simulink library "tqr"  (R2021b)
settings: Solver=VariableStepAuto  StartTime=0.0  StopTime=10.0  RelTol=1e-3
undefined symbols (not defined in the file or in its folder): ATQR_AltRDCActiveFEDUInc_X_pct, ATQR_AltRDCActiveFEDUInc_Y_enum, ATQR_AltRDCActiveFEDUTs_X_pct, ATQR_AltRDCActiveFEDUTs_Y_enum, ATQR_AltRDCActiveREDUInc_X_pct, ATQR_AltRDCActiveREDUInc_Y_enum, ATQR_AltRDCActiveREDUTs_X_pct, ATQR_AltRDCActiveREDUTs_Y_enum, ATQR_CreepFEDUTqIncSR_X_rpm, ATQR_CreepFEDUTqIncSR_Y_Nm, ATQR_CreepFEDUTs_X_rpm, ATQR_CreepFEDUTs_Y_Nm, ATQR_EcoTqFrIncGain_X_Nm, ATQR_EcoTqFrIncGain_Y_pct, ATQR_EcoTqRrIncGain_X_Nm, ATQR_EcoTqRrIncGain_Y_pct, ATQR_EL1FEDUTqDecSR_Y_Nm, ATQR_EL1FEDUTqIncSR_X_rpm, ATQR_EL1FEDUTqIncSR_Y_pct, ATQR_EL1FEDUTs_X_rpm, ATQR_EL1FEDUTs_Y_Nm, ATQR_EL1REDUTqDecSR_Y_Nm, ATQR_EL1REDUTs_Y_Nm, ATQR_FEDUEL1RegenTs_X_rpm, ATQR_FEDUTIPOutTs_X_rpm, ATQR_FrNegRateLimitIncN_X_rpm, ATQR_FrNegRateLimitIncN_Y_Nm, ATQR_FrPosRateLimitIncN_X_rpm, ATQR_FrPosRateLimitIncN_Y_Nm, ATQR_FShaftSpdTqLimCoe_X_rpm, ATQR_FTimerTqLimCoe_X_s, ATQR_FTqZeroTransUpBoundN_X_rpm, ATQR_NL1FEDUTqDecSR_Y_Nm, ATQR_NL1FEDUTqIncSR_X_rpm, ATQR_NL1FEDUTqIncSR_Y_pct, ATQR_NL1FEDUTs_X_rpm, ATQR_NL1FEDUTs_Y_Nm, ATQR_NL1REDUTqDecSR_Y_Nm, ATQR_NL1REDUTs_Y_Nm, ATQR_NormalTqFrIncGain_X_Nm, ATQR_NormalTqFrIncGain_Y_pct, ATQR_NormalTqRrIncGain_X_Nm, ATQR_NormalTqRrIncGain_Y_pct, ATQR_RrNegRateLimitIncN_X_rpm, ATQR_RrNegRateLimitIncN_Y_Nm, ATQR_RrPosRateLimitIncN_X_rpm, ATQR_RrPosRateLimitIncN_Y_Nm, ATQR_RShaftSpdTqLimCoe_X_rpm, ATQR_RTimerTqLimCoe_X_s, ATQR_SL1FEDUTqDecSR_Y_Nm, ATQR_SL1FEDUTqIncSR_X_rpm, ATQR_SL1FEDUTqIncSR_Y_pct, ATQR_SL1FEDUTs_X_rpm, ATQR_SL1FEDUTs_Y_Nm, ATQR_SL1REDUTqDecSR_Y_Nm, ATQR_SL1REDUTs_Y_Nm, ATQR_SportTqFrIncGain_X_Nm, ATQR_SportTqFrIncGain_Y_pct, ATQR_SportTqRrIncGain_X_Nm, ATQR_SportTqRrIncGain_Y_pct ... (+269)
libraries: hcu_lib x15, simulink x13, $bdroot x3
(part 9 of 9)

== system tqr/TQR/Determine Torque Request/TorqueArbitrament/TorqueSmooth/Rear wheel rate limit determination/VTQR_ECOREDURateLimitInc_Nm/LV4 ==
  VDHP_ActAPSPosn_pct : Inport
  VTQD_TqTargetShaftSpd_rpm : Inport  Port=2
  VTQR_EcoTqRrIncGain_c : Inport  Port=3
  Action Port : ActionPort
  MTQR_EL4REDUTqIncSR_Z_Nm : Lookup_n-D  BreakpointsForDimension1=ATQR_EL1FEDUTqIncSR_Y_pct  BreakpointsForDimension2=ATQR_EL1FEDUTqIncSR_X_rpm  Table=MTQR_EL4REDUTqIncSR_Z_Nm  ExtrapMethod=Clip  InternalRulePriority=Speed  RndMeth=Simplest  InputSameDT=on
      settings: InputPortMap=u0,u1
  Product : Product
  VTQR_EL4REDUTqIncSR_Nm : Outport
  wires:
  VDHP_ActAPSPosn_pct/1 -> MTQR_EL4REDUTqIncSR_Z_Nm/1
  VTQD_TqTargetShaftSpd_rpm/1 -> MTQR_EL4REDUTqIncSR_Z_Nm/2
  VTQR_EcoTqRrIncGain_c/1 -> Product/2
  MTQR_EL4REDUTqIncSR_Z_Nm/1 -> Product/1
  Product/1 -> VTQR_EL4REDUTqIncSR_Nm/1

== system tqr/TQR/Determine Torque Request/TorqueArbitrament/TorqueSmooth/Rear wheel rate limit determination/VTQR_ECOREDURateLimitInc_Nm/LV5 ==
  VDHP_ActAPSPosn_pct : Inport
  VTQD_TqTargetShaftSpd_rpm : Inport  Port=2
  VTQR_EcoTqRrIncGain_c : Inport  Port=3
  Action Port : ActionPort
  MTQR_EL5REDUTqIncSR_Z_Nm : Lookup_n-D  BreakpointsForDimension1=ATQR_EL1FEDUTqIncSR_Y_pct  BreakpointsForDimension2=ATQR_EL1FEDUTqIncSR_X_rpm  Table=MTQR_EL5REDUTqIncSR_Z_Nm  ExtrapMethod=Clip  InternalRulePriority=Speed  RndMeth=Simplest  InputSameDT=on
      settings: InputPortMap=u0,u1
  Product : Product
  VTQR_EL5REDUTqIncSR_Nm : Outport
  wires:
  VDHP_ActAPSPosn_pct/1 -> MTQR_EL5REDUTqIncSR_Z_Nm/1
  VTQD_TqTargetShaftSpd_rpm/1 -> MTQR_EL5REDUTqIncSR_Z_Nm/2
  VTQR_EcoTqRrIncGain_c/1 -> Product/2
  MTQR_EL5REDUTqIncSR_Z_Nm/1 -> Product/1
  Product/1 -> VTQR_EL5REDUTqIncSR_Nm/1

== system tqr/TQR/Determine Torque Request/TorqueArbitrament/TorqueSmooth/Rear wheel rate limit determination/VTQR_ECOREDURateLimitInc_Nm/OPD ==
  VDHP_ActAPSPosn_pct : Inport
  VTQD_TqTargetShaftSpd_rpm : Inport  Port=2
  VTQR_EcoTqRrIncGain_c : Inport  Port=3
  Action Port : ActionPort
  MTQR_EOPDREDUTqIncSR_Z_Nm : Lookup_n-D  BreakpointsForDimension1=ATQR_EL1FEDUTqIncSR_Y_pct  BreakpointsForDimension2=ATQR_EL1FEDUTqIncSR_X_rpm  Table=MTQR_EOPDREDUTqIncSR_Z_Nm  ExtrapMethod=Clip  InternalRulePriority=Speed  RndMeth=Simplest  InputSameDT=on
      settings: InputPortMap=u0,u1
  Product : Product
  VTQR_EOPDREDUTqIncSR_Nm : Outport
  wires:
  VDHP_ActAPSPosn_pct/1 -> MTQR_EOPDREDUTqIncSR_Z_Nm/1
  VTQD_TqTargetShaftSpd_rpm/1 -> MTQR_EOPDREDUTqIncSR_Z_Nm/2
  VTQR_EcoTqRrIncGain_c/1 -> Product/2
  MTQR_EOPDREDUTqIncSR_Z_Nm/1 -> Product/1
  Product/1 -> VTQR_EOPDREDUTqIncSR_Nm/1

== system tqr/TQR/Determine Torque Request/TorqueArbitrament/TorqueSmooth/Rear wheel rate limit determination/VTQR_NORMALREDURateLimitDec_Nm/Invalid ==
  VTQR_REDUWhlTqReqSmoothDelay_Nm : Inport
  VTQD_TqTargetShaftSpd_rpm : Inport  Port=2
  Action Port : ActionPort
  MTQR_NL1REDUTqDecSR_Z_Nm : Lookup_n-D  BreakpointsForDimension1=ATQR_NL1REDUTqDecSR_Y_Nm  BreakpointsForDimension2=ATQR_NL1FEDUTqIncSR_X_rpm  Table=MTQR_NL1REDUTqDecSR_Z_Nm  ExtrapMethod=Clip  InternalRulePriority=Speed  RndMeth=Simplest  InputSameDT=on
      settings: InputPortMap=u0,u1
  VTQR_NL1REDUTqDecSR_Nm : Outport
  wires:
  VTQD_TqTargetShaftSpd_rpm/1 -> MTQR_NL1REDUTqDecSR_Z_Nm/2
  MTQR_NL1REDUTqDecSR_Z_Nm/1 -> VTQR_NL1REDUTqDecSR_Nm/1
  VTQR_REDUWhlTqReqSmoothDelay_Nm/1 -> MTQR_NL1REDUTqDecSR_Z_Nm/1

== system tqr/TQR/Determine Torque Request/TorqueArbitrament/TorqueSmooth/Rear wheel rate limit determination/VTQR_NORMALREDURateLimitDec_Nm/LV1 ==
  VTQR_REDUWhlTqReqSmoothDelay_Nm : Inport
  VTQD_TqTargetShaftSpd_rpm : Inport  Port=2
  Action Port : ActionPort
  MTQR_NL1REDUTqDecSR_Z_Nm : Lookup_n-D  BreakpointsForDimension1=ATQR_NL1REDUTqDecSR_Y_Nm  BreakpointsForDimension2=ATQR_NL1FEDUTqIncSR_X_rpm  Table=MTQR_NL1REDUTqDecSR_Z_Nm  ExtrapMethod=Clip  InternalRulePriority=Speed  RndMeth=Simplest  InputSameDT=on
      settings: InputPortMap=u0,u1
  VTQR_NL1REDUTqDecSR_Nm : Outport
  wires:
  VTQR_REDUWhlTqReqSmoothDelay_Nm/1 -> MTQR_NL1REDUTqDecSR_Z_Nm/1
  MTQR_NL1REDUTqDecSR_Z_Nm/1 -> VTQR_NL1REDUTqDecSR_Nm/1
  VTQD_TqTargetShaftSpd_rpm/1 -> MTQR_NL1REDUTqDecSR_Z_Nm/2

== system tqr/TQR/Determine Torque Request/TorqueArbitrament/TorqueSmooth/Rear wheel rate limit determination/VTQR_NORMALREDURateLimitDec_Nm/LV2 ==
  VTQR_REDUWhlTqReqSmoothDelay_Nm : Inport
  VTQD_TqTargetShaftSpd_rpm : Inport  Port=2
  Action Port : ActionPort
  MTQR_NL2REDUTqDecSR_Z_Nm : Lookup_n-D  BreakpointsForDimension1=ATQR_NL1REDUTqDecSR_Y_Nm  BreakpointsForDimension2=ATQR_NL1FEDUTqIncSR_X_rpm  Table=MTQR_NL2REDUTqDecSR_Z_Nm  ExtrapMethod=Clip  InternalRulePriority=Speed  RndMeth=Simplest  InputSameDT=on
      settings: InputPortMap=u0,u1
  VTQR_NL2REDUTqDecSR_Nm : Outport
  wires:
  MTQR_NL2REDUTqDecSR_Z_Nm/1 -> VTQR_NL2REDUTqDecSR_Nm/1
  VTQR_REDUWhlTqReqSmoothDelay_Nm/1 -> MTQR_NL2REDUTqDecSR_Z_Nm/1
  VTQD_TqTargetShaftSpd_rpm/1 -> MTQR_NL2REDUTqDecSR_Z_Nm/2

== system tqr/TQR/Determine Torque Request/TorqueArbitrament/TorqueSmooth/Rear wheel rate limit determination/VTQR_NORMALREDURateLimitDec_Nm/LV3 ==
  VTQR_REDUWhlTqReqSmoothDelay_Nm : Inport
  VTQD_TqTargetShaftSpd_rpm : Inport  Port=2
  Action Port : ActionPort
  MTQR_NL3REDUTqDecSR_Z_Nm : Lookup_n-D  BreakpointsForDimension1=ATQR_NL1REDUTqDecSR_Y_Nm  BreakpointsForDimension2=ATQR_NL1FEDUTqIncSR_X_rpm  Table=MTQR_NL3REDUTqDecSR_Z_Nm  ExtrapMethod=Clip  InternalRulePriority=Speed  RndMeth=Simplest  InputSameDT=on
      settings: InputPortMap=u0,u1
  VTQR_NL3REDUTqDecSR_Nm : Outport
  wires:
  VTQR_REDUWhlTqReqSmoothDelay_Nm/1 -> MTQR_NL3REDUTqDecSR_Z_Nm/1
  VTQD_TqTargetShaftSpd_rpm/1 -> MTQR_NL3REDUTqDecSR_Z_Nm/2
  MTQR_NL3REDUTqDecSR_Z_Nm/1 -> VTQR_NL3REDUTqDecSR_Nm/1

== system tqr/TQR/Determine Torque Request/TorqueArbitrament/TorqueSmooth/Rear wheel rate limit determination/VTQR_NORMALREDURateLimitDec_Nm/LV4 ==
  VTQR_REDUWhlTqReqSmoothDelay_Nm : Inport
  VTQD_TqTargetShaftSpd_rpm : Inport  Port=2
  Action Port : ActionPort
  MTQR_NL4REDUTqDecSR_Z_Nm : Lookup_n-D  BreakpointsForDimension1=ATQR_NL1REDUTqDecSR_Y_Nm  BreakpointsForDimension2=ATQR_NL1FEDUTqIncSR_X_rpm  Table=MTQR_NL4REDUTqDecSR_Z_Nm  ExtrapMethod=Clip  InternalRulePriority=Speed  RndMeth=Simplest  InputSameDT=on
      settings: InputPortMap=u0,u1
  VTQR_NL4REDUTqDecSR_Nm : Outport
  wires:
  VTQR_REDUWhlTqReqSmoothDelay_Nm/1 -> MTQR_NL4REDUTqDecSR_Z_Nm/1
  VTQD_TqTargetShaftSpd_rpm/1 -> MTQR_NL4REDUTqDecSR_Z_Nm/2
  MTQR_NL4REDUTqDecSR_Z_Nm/1 -> VTQR_NL4REDUTqDecSR_Nm/1

== system tqr/TQR/Determine Torque Request/TorqueArbitrament/TorqueSmooth/Rear wheel rate limit determination/VTQR_NORMALREDURateLimitDec_Nm/LV5 ==
  VTQR_REDUWhlTqReqSmoothDelay_Nm : Inport
  VTQD_TqTargetShaftSpd_rpm : Inport  Port=2
  Action Port : ActionPort
  MTQR_NL5REDUTqDecSR_Z_Nm : Lookup_n-D  BreakpointsForDimension1=ATQR_NL1REDUTqDecSR_Y_Nm  BreakpointsForDimension2=ATQR_NL1FEDUTqIncSR_X_rpm  Table=MTQR_NL5REDUTqDecSR_Z_Nm  ExtrapMethod=Clip  InternalRulePriority=Speed  RndMeth=Simplest  InputSameDT=on
      settings: InputPortMap=u0,u1
  VTQR_NL5REDUTqDecSR_Nm : Outport
  wires:
  VTQR_REDUWhlTqReqSmoothDelay_Nm/1 -> MTQR_NL5REDUTqDecSR_Z_Nm/1
  VTQD_TqTargetShaftSpd_rpm/1 -> MTQR_NL5REDUTqDecSR_Z_Nm/2
  MTQR_NL5REDUTqDecSR_Z_Nm/1 -> VTQR_NL5REDUTqDecSR_Nm/1

== system tqr/TQR/Determine Torque Request/TorqueArbitrament/TorqueSmooth/Rear wheel rate limit determination/VTQR_NORMALREDURateLimitDec_Nm/OPD ==
  VTQR_REDUWhlTqReqSmoothDelay_Nm : Inport
  VTQD_TqTargetShaftSpd_rpm : Inport  Port=2
  Action Port : ActionPort
  MTQR_NOPDREDUTqDecSR_Z_Nm : Lookup_n-D  BreakpointsForDimension1=ATQR_NL1REDUTqDecSR_Y_Nm  BreakpointsForDimension2=ATQR_NL1FEDUTqIncSR_X_rpm  Table=MTQR_NOPDREDUTqDecSR_Z_Nm  ExtrapMethod=Clip  InternalRulePriority=Speed  RndMeth=Simplest  InputSameDT=on
      settings: InputPortMap=u0,u1
  VTQR_NOPDREDUTqDecSR_Nm : Outport
  wires:
  VTQR_REDUWhlTqReqSmoothDelay_Nm/1 -> MTQR_NOPDREDUTqDecSR_Z_Nm/1
  VTQD_TqTargetShaftSpd_rpm/1 -> MTQR_NOPDREDUTqDecSR_Z_Nm/2
  MTQR_NOPDREDUTqDecSR_Z_Nm/1 -> VTQR_NOPDREDUTqDecSR_Nm/1

== system tqr/TQR/Determine Torque Request/TorqueArbitrament/TorqueSmooth/Rear wheel rate limit determination/VTQR_NORMALREDURateLimitInc_Nm/Invalid ==
  VDHP_ActAPSPosn_pct : Inport
  VTQD_TqTargetShaftSpd_rpm : Inport  Port=2
  Action Port : ActionPort
  MTQR_NL1REDUTqIncSR_Z_Nm : Lookup_n-D  BreakpointsForDimension1=ATQR_NL1FEDUTqIncSR_Y_pct  BreakpointsForDimension2=ATQR_NL1FEDUTqIncSR_X_rpm  Table=MTQR_NL1REDUTqIncSR_Z_Nm  ExtrapMethod=Clip  InternalRulePriority=Speed  RndMeth=Simplest  InputSameDT=on
      settings: InputPortMap=u0,u1
  VTQR_NL1REDUTqIncSR_Nm : Outport
  wires:
  VTQD_TqTargetShaftSpd_rpm/1 -> MTQR_NL1REDUTqIncSR_Z_Nm/2
  MTQR_NL1REDUTqIncSR_Z_Nm/1 -> VTQR_NL1REDUTqIncSR_Nm/1
  VDHP_ActAPSPosn_pct/1 -> MTQR_NL1REDUTqIncSR_Z_Nm/1

== system tqr/TQR/Determine Torque Request/TorqueArbitrament/TorqueSmooth/Rear wheel rate limit determination/VTQR_NORMALREDURateLimitInc_Nm/LV1 ==
  VDHP_ActAPSPosn_pct : Inport
  VTQD_TqTargetShaftSpd_rpm : Inport  Port=2
  VTQR_NormalTqRrIncGain_c : Inport  Port=3
  Action Port : ActionPort
  MTQR_NL1REDUTqIncSR_Z_Nm : Lookup_n-D  BreakpointsForDimension1=ATQR_NL1FEDUTqIncSR_Y_pct  BreakpointsForDimension2=ATQR_NL1FEDUTqIncSR_X_rpm  Table=MTQR_NL1REDUTqIncSR_Z_Nm  ExtrapMethod=Clip  InternalRulePriority=Speed  RndMeth=Simplest  InputSameDT=on
      settings: InputPortMap=u0,u1
  Product : Product
  VTQR_NL1REDUTqIncSR_Nm : Outport
  wires:
  VDHP_ActAPSPosn_pct/1 -> MTQR_NL1REDUTqIncSR_Z_Nm/1
  VTQD_TqTargetShaftSpd_rpm/1 -> MTQR_NL1REDUTqIncSR_Z_Nm/2
  MTQR_NL1REDUTqIncSR_Z_Nm/1 -> Product/1
  Product/1 -> VTQR_NL1REDUTqIncSR_Nm/1
  VTQR_NormalTqRrIncGain_c/1 -> Product/2

== system tqr/TQR/Determine Torque Request/TorqueArbitrament/TorqueSmooth/Rear wheel rate limit determination/VTQR_NORMALREDURateLimitInc_Nm/LV2 ==
  VDHP_ActAPSPosn_pct : Inport
  VTQD_TqTargetShaftSpd_rpm : Inport  Port=2
  VTQR_NormalTqRrIncGain_c : Inport  Port=3
  Action Port : ActionPort
  MTQR_NL2REDUTqIncSR_Z_Nm : Lookup_n-D  BreakpointsForDimension1=ATQR_NL1FEDUTqIncSR_Y_pct  BreakpointsForDimension2=ATQR_NL1FEDUTqIncSR_X_rpm  Table=MTQR_NL2REDUTqIncSR_Z_Nm  ExtrapMethod=Clip  InternalRulePriority=Speed  RndMeth=Simplest  InputSameDT=on
      settings: InputPortMap=u0,u1
  Product : Product
  VTQR_NL2REDUTqIncSR_Nm : Outport
  wires:
  VDHP_ActAPSPosn_pct/1 -> MTQR_NL2REDUTqIncSR_Z_Nm/1
  VTQD_TqTargetShaftSpd_rpm/1 -> MTQR_NL2REDUTqIncSR_Z_Nm/2
  Product/1 -> VTQR_NL2REDUTqIncSR_Nm/1
  MTQR_NL2REDUTqIncSR_Z_Nm/1 -> Product/1
  VTQR_NormalTqRrIncGain_c/1 -> Product/2

== system tqr/TQR/Determine Torque Request/TorqueArbitrament/TorqueSmooth/Rear wheel rate limit determination/VTQR_NORMALREDURateLimitInc_Nm/LV3 ==
  VDHP_ActAPSPosn_pct : Inport
  VTQD_TqTargetShaftSpd_rpm : Inport  Port=2
  VTQR_NormalTqRrIncGain_c : Inport  Port=3
  Action Port : ActionPort
  MTQR_NL3REDUTqIncSR_Z_Nm : Lookup_n-D  BreakpointsForDimension1=ATQR_NL1FEDUTqIncSR_Y_pct  BreakpointsForDimension2=ATQR_NL1FEDUTqIncSR_X_rpm  Table=MTQR_NL3REDUTqIncSR_Z_Nm  ExtrapMethod=Clip  InternalRulePriority=Speed  RndMeth=Simplest  InputSameDT=on
      settings: InputPortMap=u0,u1
  Product : Product
  VTQR_NL3REDUTqIncSR_Nm : Outport
  wires:
  VDHP_ActAPSPosn_pct/1 -> MTQR_NL3REDUTqIncSR_Z_Nm/1
  VTQD_TqTargetShaftSpd_rpm/1 -> MTQR_NL3REDUTqIncSR_Z_Nm/2
  Product/1 -> VTQR_NL3REDUTqIncSR_Nm/1
  MTQR_NL3REDUTqIncSR_Z_Nm/1 -> Product/1
  VTQR_NormalTqRrIncGain_c/1 -> Product/2

== system tqr/TQR/Determine Torque Request/TorqueArbitrament/TorqueSmooth/Rear wheel rate limit determination/VTQR_NORMALREDURateLimitInc_Nm/LV4 ==
  VDHP_ActAPSPosn_pct : Inport
  VTQD_TqTargetShaftSpd_rpm : Inport  Port=2
  VTQR_NormalTqRrIncGain_c : Inport  Port=3
  Action Port : ActionPort
  MTQR_NL4REDUTqIncSR_Z_Nm : Lookup_n-D  BreakpointsForDimension1=ATQR_NL1FEDUTqIncSR_Y_pct  BreakpointsForDimension2=ATQR_NL1FEDUTqIncSR_X_rpm  Table=MTQR_NL4REDUTqIncSR_Z_Nm  ExtrapMethod=Clip  InternalRulePriority=Speed  RndMeth=Simplest  InputSameDT=on
      settings: InputPortMap=u0,u1
  Product : Product
  VTQR_NL4REDUTqIncSR_Nm : Outport
  wires:
  VDHP_ActAPSPosn_pct/1 -> MTQR_NL4REDUTqIncSR_Z_Nm/1
  VTQD_TqTargetShaftSpd_rpm/1 -> MTQR_NL4REDUTqIncSR_Z_Nm/2
  VTQR_NormalTqRrIncGain_c/1 -> Product/2
  Product/1 -> VTQR_NL4REDUTqIncSR_Nm/1
  MTQR_NL4REDUTqIncSR_Z_Nm/1 -> Product/1

== system tqr/TQR/Determine Torque Request/TorqueArbitrament/TorqueSmooth/Rear wheel rate limit determination/VTQR_NORMALREDURateLimitInc_Nm/LV5 ==
  VDHP_ActAPSPosn_pct : Inport
  VTQD_TqTargetShaftSpd_rpm : Inport  Port=2
  VTQR_NormalTqRrIncGain_c : Inport  Port=3
  Action Port : ActionPort
  MTQR_NL5REDUTqIncSR_Z_Nm : Lookup_n-D  BreakpointsForDimension1=ATQR_NL1FEDUTqIncSR_Y_pct  BreakpointsForDimension2=ATQR_NL1FEDUTqIncSR_X_rpm  Table=MTQR_NL5REDUTqIncSR_Z_Nm  ExtrapMethod=Clip  InternalRulePriority=Speed  RndMeth=Simplest  InputSameDT=on
      settings: InputPortMap=u0,u1
  Product : Product
  VTQR_NL5REDUTqIncSR_Nm : Outport
  wires:
  VDHP_ActAPSPosn_pct/1 -> MTQR_NL5REDUTqIncSR_Z_Nm/1
  VTQD_TqTargetShaftSpd_rpm/1 -> MTQR_NL5REDUTqIncSR_Z_Nm/2
  Product/1 -> VTQR_NL5REDUTqIncSR_Nm/1
  MTQR_NL5REDUTqIncSR_Z_Nm/1 -> Product/1
  VTQR_NormalTqRrIncGain_c/1 -> Product/2

== system tqr/TQR/Determine Torque Request/TorqueArbitrament/TorqueSmooth/Rear wheel rate limit determination/VTQR_NORMALREDURateLimitInc_Nm/OPD ==
  VDHP_ActAPSPosn_pct : Inport
  VTQD_TqTargetShaftSpd_rpm : Inport  Port=2
  VTQR_NormalTqRrIncGain_c : Inport  Port=3
  Action Port : ActionPort
  MTQR_NOPDREDUTqIncSR_Z_Nm : Lookup_n-D  BreakpointsForDimension1=ATQR_NL1FEDUTqIncSR_Y_pct  BreakpointsForDimension2=ATQR_NL1FEDUTqIncSR_X_rpm  Table=MTQR_NOPDREDUTqIncSR_Z_Nm  ExtrapMethod=Clip  InternalRulePriority=Speed  RndMeth=Simplest  InputSameDT=on
      settings: InputPortMap=u0,u1
  Product : Product
  VTQR_NOPDREDUTqIncSR_Nm : Outport
  wires:
  VDHP_ActAPSPosn_pct/1 -> MTQR_NOPDREDUTqIncSR_Z_Nm/1
  VTQD_TqTargetShaftSpd_rpm/1 -> MTQR_NOPDREDUTqIncSR_Z_Nm/2
  MTQR_NOPDREDUTqIncSR_Z_Nm/1 -> Product/1
  Product/1 -> VTQR_NOPDREDUTqIncSR_Nm/1
  VTQR_NormalTqRrIncGain_c/1 -> Product/2

== system tqr/TQR/Determine Torque Request/TorqueArbitrament/TorqueSmooth/Rear wheel rate limit determination/VTQR_SPORTREDURateLimitDec_Nm/Invalid ==
  VTQR_REDUWhlTqReqSmoothDelay_Nm : Inport
  VTQD_TqTargetShaftSpd_rpm : Inport  Port=2
  Action Port : ActionPort
  MTQR_SL1REDUTqDecSR_Z_Nm : Lookup_n-D  BreakpointsForDimension1=ATQR_SL1REDUTqDecSR_Y_Nm  BreakpointsForDimension2=ATQR_SL1FEDUTqIncSR_X_rpm  Table=MTQR_SL1REDUTqDecSR_Z_Nm  ExtrapMethod=Clip  InternalRulePriority=Speed  RndMeth=Simplest  InputSameDT=on
      settings: InputPortMap=u0,u1
  VTQR_SL1REDUTqDecSR_Nm : Outport
  wires:
  VTQD_TqTargetShaftSpd_rpm/1 -> MTQR_SL1REDUTqDecSR_Z_Nm/2
  MTQR_SL1REDUTqDecSR_Z_Nm/1 -> VTQR_SL1REDUTqDecSR_Nm/1
  VTQR_REDUWhlTqReqSmoothDelay_Nm/1 -> MTQR_SL1REDUTqDecSR_Z_Nm/1

== system tqr/TQR/Determine Torque Request/TorqueArbitrament/TorqueSmooth/Rear wheel rate limit determination/VTQR_SPORTREDURateLimitDec_Nm/LV1 ==
  VTQR_REDUWhlTqReqSmoothDelay_Nm : Inport
  VTQD_TqTargetShaftSpd_rpm : Inport  Port=2
  Action Port : ActionPort
  MTQR_SL1REDUTqDecSR_Z_Nm : Lookup_n-D  BreakpointsForDimension1=ATQR_SL1REDUTqDecSR_Y_Nm  BreakpointsForDimension2=ATQR_SL1FEDUTqIncSR_X_rpm  Table=MTQR_SL1REDUTqDecSR_Z_Nm  ExtrapMethod=Clip  InternalRulePriority=Speed  RndMeth=Simplest  InputSameDT=on
      settings: InputPortMap=u0,u1
  VTQR_SL1REDUTqDecSR_Nm : Outport
  wires:
  VTQR_REDUWhlTqReqSmoothDelay_Nm/1 -> MTQR_SL1REDUTqDecSR_Z_Nm/1
  MTQR_SL1REDUTqDecSR_Z_Nm/1 -> VTQR_SL1REDUTqDecSR_Nm/1
  VTQD_TqTargetShaftSpd_rpm/1 -> MTQR_SL1REDUTqDecSR_Z_Nm/2

== system tqr/TQR/Determine Torque Request/TorqueArbitrament/TorqueSmooth/Rear wheel rate limit determination/VTQR_SPORTREDURateLimitDec_Nm/LV2 ==
  VTQR_REDUWhlTqReqSmoothDelay_Nm : Inport
  VTQD_TqTargetShaftSpd_rpm : Inport  Port=2
  Action Port : ActionPort
  MTQR_SL2REDUTqDecSR_Z_Nm : Lookup_n-D  BreakpointsForDimension1=ATQR_SL1REDUTqDecSR_Y_Nm  BreakpointsForDimension2=ATQR_SL1FEDUTqIncSR_X_rpm  Table=MTQR_SL2REDUTqDecSR_Z_Nm  ExtrapMethod=Clip  InternalRulePriority=Speed  RndMeth=Simplest  InputSameDT=on
      settings: InputPortMap=u0,u1
  VTQR_SL2REDUTqDecSR_Nm : Outport
  wires:
  MTQR_SL2REDUTqDecSR_Z_Nm/1 -> VTQR_SL2REDUTqDecSR_Nm/1
  VTQR_REDUWhlTqReqSmoothDelay_Nm/1 -> MTQR_SL2REDUTqDecSR_Z_Nm/1
  VTQD_TqTargetShaftSpd_rpm/1 -> MTQR_SL2REDUTqDecSR_Z_Nm/2

== system tqr/TQR/Determine Torque Request/TorqueArbitrament/TorqueSmooth/Rear wheel rate limit determination/VTQR_SPORTREDURateLimitDec_Nm/LV3 ==
  VTQR_REDUWhlTqReqSmoothDelay_Nm : Inport
  VTQD_TqTargetShaftSpd_rpm : Inport  Port=2
  Action Port : ActionPort
  MTQR_SL3REDUTqDecSR_Z_Nm : Lookup_n-D  BreakpointsForDimension1=ATQR_SL1REDUTqDecSR_Y_Nm  BreakpointsForDimension2=ATQR_SL1FEDUTqIncSR_X_rpm  Table=MTQR_SL3REDUTqDecSR_Z_Nm  ExtrapMethod=Clip  InternalRulePriority=Speed  RndMeth=Simplest  InputSameDT=on
      settings: InputPortMap=u0,u1
  VTQR_SL3REDUTqDecSR_Nm : Outport
  wires:
  VTQR_REDUWhlTqReqSmoothDelay_Nm/1 -> MTQR_SL3REDUTqDecSR_Z_Nm/1
  VTQD_TqTargetShaftSpd_rpm/1 -> MTQR_SL3REDUTqDecSR_Z_Nm/2
  MTQR_SL3REDUTqDecSR_Z_Nm/1 -> VTQR_SL3REDUTqDecSR_Nm/1

== system tqr/TQR/Determine Torque Request/TorqueArbitrament/TorqueSmooth/Rear wheel rate limit determination/VTQR_SPORTREDURateLimitDec_Nm/LV4 ==
  VTQR_REDUWhlTqReqSmoothDelay_Nm : Inport
  VTQD_TqTargetShaftSpd_rpm : Inport  Port=2
  Action Port : ActionPort
  MTQR_SL4REDUTqDecSR_Z_Nm : Lookup_n-D  BreakpointsForDimension1=ATQR_SL1REDUTqDecSR_Y_Nm  BreakpointsForDimension2=ATQR_SL1FEDUTqIncSR_X_rpm  Table=MTQR_SL4REDUTqDecSR_Z_Nm  ExtrapMethod=Clip  InternalRulePriority=Speed  RndMeth=Simplest  InputSameDT=on
      settings: InputPortMap=u0,u1
  VTQR_SL4REDUTqDecSR_Nm : Outport
  wires:
  VTQR_REDUWhlTqReqSmoothDelay_Nm/1 -> MTQR_SL4REDUTqDecSR_Z_Nm/1
  VTQD_TqTargetShaftSpd_rpm/1 -> MTQR_SL4REDUTqDecSR_Z_Nm/2
  MTQR_SL4REDUTqDecSR_Z_Nm/1 -> VTQR_SL4REDUTqDecSR_Nm/1

== system tqr/TQR/Determine Torque Request/TorqueArbitrament/TorqueSmooth/Rear wheel rate limit determination/VTQR_SPORTREDURateLimitDec_Nm/LV5 ==
  VTQR_REDUWhlTqReqSmoothDelay_Nm : Inport
  VTQD_TqTargetShaftSpd_rpm : Inport  Port=2
  Action Port : ActionPort
  MTQR_SL5REDUTqDecSR_Z_Nm : Lookup_n-D  BreakpointsForDimension1=ATQR_SL1REDUTqDecSR_Y_Nm  BreakpointsForDimension2=ATQR_SL1FEDUTqIncSR_X_rpm  Table=MTQR_SL5REDUTqDecSR_Z_Nm  ExtrapMethod=Clip  InternalRulePriority=Speed  RndMeth=Simplest  InputSameDT=on
      settings: InputPortMap=u0,u1
  VTQR_SL5REDUTqIDecSR_Nm : Outport
  wires:
  VTQR_REDUWhlTqReqSmoothDelay_Nm/1 -> MTQR_SL5REDUTqDecSR_Z_Nm/1
  VTQD_TqTargetShaftSpd_rpm/1 -> MTQR_SL5REDUTqDecSR_Z_Nm/2
  MTQR_SL5REDUTqDecSR_Z_Nm/1 -> VTQR_SL5REDUTqIDecSR_Nm/1

== system tqr/TQR/Determine Torque Request/TorqueArbitrament/TorqueSmooth/Rear wheel rate limit determination/VTQR_SPORTREDURateLimitDec_Nm/OPD ==
  VTQR_REDUWhlTqReqSmoothDelay_Nm : Inport
  VTQD_TqTargetShaftSpd_rpm : Inport  Port=2
  Action Port : ActionPort
  MTQR_SOPDREDUTqDecSR_Z_Nm : Lookup_n-D  BreakpointsForDimension1=ATQR_SL1REDUTqDecSR_Y_Nm  BreakpointsForDimension2=ATQR_SL1FEDUTqIncSR_X_rpm  Table=MTQR_SOPDREDUTqDecSR_Z_Nm  ExtrapMethod=Clip  InternalRulePriority=Speed  RndMeth=Simplest  InputSameDT=on
      settings: InputPortMap=u0,u1
  VTQR_SOPDREDUTqDecSR_Nm : Outport
  wires:
  VTQR_REDUWhlTqReqSmoothDelay_Nm/1 -> MTQR_SOPDREDUTqDecSR_Z_Nm/1
  VTQD_TqTargetShaftSpd_rpm/1 -> MTQR_SOPDREDUTqDecSR_Z_Nm/2
  MTQR_SOPDREDUTqDecSR_Z_Nm/1 -> VTQR_SOPDREDUTqDecSR_Nm/1

== system tqr/TQR/Determine Torque Request/TorqueArbitrament/TorqueSmooth/Rear wheel rate limit determination/VTQR_SPORTREDURateLimitInc_Nm/Invalid ==
  VDHP_ActAPSPosn_pct : Inport
  VTQD_TqTargetShaftSpd_rpm : Inport  Port=2
  Action Port : ActionPort
  MTQR_SL1REDUTqIncSR_Z_Nm : Lookup_n-D  BreakpointsForDimension1=ATQR_SL1FEDUTqIncSR_Y_pct  BreakpointsForDimension2=ATQR_SL1FEDUTqIncSR_X_rpm  Table=MTQR_SL1REDUTqIncSR_Z_Nm  ExtrapMethod=Clip  InternalRulePriority=Speed  RndMeth=Simplest  InputSameDT=on
      settings: InputPortMap=u0,u1
  VTQR_SL1REDUTqIncSR_Nm : Outport
  wires:
  VDHP_ActAPSPosn_pct/1 -> MTQR_SL1REDUTqIncSR_Z_Nm/1
  MTQR_SL1REDUTqIncSR_Z_Nm/1 -> VTQR_SL1REDUTqIncSR_Nm/1
  VTQD_TqTargetShaftSpd_rpm/1 -> MTQR_SL1REDUTqIncSR_Z_Nm/2

== system tqr/TQR/Determine Torque Request/TorqueArbitrament/TorqueSmooth/Rear wheel rate limit determination/VTQR_SPORTREDURateLimitInc_Nm/LV1 ==
  VDHP_ActAPSPosn_pct : Inport
  VTQD_TqTargetShaftSpd_rpm : Inport  Port=2
  VTQR_SportTqRrIncGain_c : Inport  Port=3
  Action Port : ActionPort
  MTQR_SL1REDUTqIncSR_Z_Nm : Lookup_n-D  BreakpointsForDimension1=ATQR_SL1FEDUTqIncSR_Y_pct  BreakpointsForDimension2=ATQR_SL1FEDUTqIncSR_X_rpm  Table=MTQR_SL1REDUTqIncSR_Z_Nm  ExtrapMethod=Clip  InternalRulePriority=Speed  RndMeth=Simplest  InputSameDT=on
      settings: InputPortMap=u0,u1
  Product : Product
  VTQR_SL1REDUTqIncSR_Nm : Outport
  wires:
  VTQD_TqTargetShaftSpd_rpm/1 -> MTQR_SL1REDUTqIncSR_Z_Nm/2
  VDHP_ActAPSPosn_pct/1 -> MTQR_SL1REDUTqIncSR_Z_Nm/1
  MTQR_SL1REDUTqIncSR_Z_Nm/1 -> Product/1
  Product/1 -> VTQR_SL1REDUTqIncSR_Nm/1
  VTQR_SportTqRrIncGain_c/1 -> Product/2

== system tqr/TQR/Determine Torque Request/TorqueArbitrament/TorqueSmooth/Rear wheel rate limit determination/VTQR_SPORTREDURateLimitInc_Nm/LV2 ==
  VDHP_ActAPSPosn_pct : Inport
  VTQD_TqTargetShaftSpd_rpm : Inport  Port=2
  VTQR_SportTqRrIncGain_c : Inport  Port=3
  Action Port : ActionPort
  MTQR_SL2REDUTqIncSR_Z_Nm : Lookup_n-D  BreakpointsForDimension1=ATQR_SL1FEDUTqIncSR_Y_pct  BreakpointsForDimension2=ATQR_SL1FEDUTqIncSR_X_rpm  Table=MTQR_SL2REDUTqIncSR_Z_Nm  ExtrapMethod=Clip  InternalRulePriority=Speed  RndMeth=Simplest  InputSameDT=on
      settings: InputPortMap=u0,u1
  Product : Product
  VTQR_SL2REDUTqIncSR_Nm : Outport
  wires:
  VTQD_TqTargetShaftSpd_rpm/1 -> MTQR_SL2REDUTqIncSR_Z_Nm/2
  VDHP_ActAPSPosn_pct/1 -> MTQR_SL2REDUTqIncSR_Z_Nm/1
  VTQR_SportTqRrIncGain_c/1 -> Product/2
  MTQR_SL2REDUTqIncSR_Z_Nm/1 -> Product/1
  Product/1 -> VTQR_SL2REDUTqIncSR_Nm/1

== system tqr/TQR/Determine Torque Request/TorqueArbitrament/TorqueSmooth/Rear wheel rate limit determination/VTQR_SPORTREDURateLimitInc_Nm/LV3 ==
  VDHP_ActAPSPosn_pct : Inport
  VTQD_TqTargetShaftSpd_rpm : Inport  Port=2
  VTQR_SportTqRrIncGain_c : Inport  Port=3
  Action Port : ActionPort
  MTQR_SL3REDUTqIncSR_Z_Nm : Lookup_n-D  BreakpointsForDimension1=ATQR_SL1FEDUTqIncSR_Y_pct  BreakpointsForDimension2=ATQR_SL1FEDUTqIncSR_X_rpm  Table=MTQR_SL3REDUTqIncSR_Z_Nm  ExtrapMethod=Clip  InternalRulePriority=Speed  RndMeth=Simplest  InputSameDT=on
      settings: InputPortMap=u0,u1
  Product : Product
  VTQR_SL3REDUTqIncSR_Nm : Outport
  wires:
  VTQD_TqTargetShaftSpd_rpm/1 -> MTQR_SL3REDUTqIncSR_Z_Nm/2
  VDHP_ActAPSPosn_pct/1 -> MTQR_SL3REDUTqIncSR_Z_Nm/1
  VTQR_SportTqRrIncGain_c/1 -> Product/2
  MTQR_SL3REDUTqIncSR_Z_Nm/1 -> Product/1
  Product/1 -> VTQR_SL3REDUTqIncSR_Nm/1

== system tqr/TQR/Determine Torque Request/TorqueArbitrament/TorqueSmooth/Rear wheel rate limit determination/VTQR_SPORTREDURateLimitInc_Nm/LV4 ==
  VDHP_ActAPSPosn_pct : Inport
  VTQD_TqTargetShaftSpd_rpm : Inport  Port=2
  VTQR_SportTqRrIncGain_c : Inport  Port=3
  Action Port : ActionPort
  MTQR_SL4REDUTqIncSR_Z_Nm : Lookup_n-D  BreakpointsForDimension1=ATQR_SL1FEDUTqIncSR_Y_pct  BreakpointsForDimension2=ATQR_SL1FEDUTqIncSR_X_rpm  Table=MTQR_SL4REDUTqIncSR_Z_Nm  ExtrapMethod=Clip  InternalRulePriority=Speed  RndMeth=Simplest  InputSameDT=on
      settings: InputPortMap=u0,u1
  Product : Product
  VTQR_SL4REDUTqIncSR_Nm : Outport
  wires:
  VTQD_TqTargetShaftSpd_rpm/1 -> MTQR_SL4REDUTqIncSR_Z_Nm/2
  VDHP_ActAPSPosn_pct/1 -> MTQR_SL4REDUTqIncSR_Z_Nm/1
  VTQR_SportTqRrIncGain_c/1 -> Product/2
  MTQR_SL4REDUTqIncSR_Z_Nm/1 -> Product/1
  Product/1 -> VTQR_SL4REDUTqIncSR_Nm/1

== system tqr/TQR/Determine Torque Request/TorqueArbitrament/TorqueSmooth/Rear wheel rate limit determination/VTQR_SPORTREDURateLimitInc_Nm/LV5 ==
  VDHP_ActAPSPosn_pct : Inport
  VTQD_TqTargetShaftSpd_rpm : Inport  Port=2
  VTQR_SportTqRrIncGain_c : Inport  Port=3
  Action Port : ActionPort
  MTQR_SL5REDUTqIncSR_Z_Nm : Lookup_n-D  BreakpointsForDimension1=ATQR_SL1FEDUTqIncSR_Y_pct  BreakpointsForDimension2=ATQR_SL1FEDUTqIncSR_X_rpm  Table=MTQR_SL5REDUTqIncSR_Z_Nm  ExtrapMethod=Clip  InternalRulePriority=Speed  RndMeth=Simplest  InputSameDT=on
      settings: InputPortMap=u0,u1
  Product : Product
  VTQR_SL5REDUTqIncSR_Nm : Outport
  wires:
  VTQD_TqTargetShaftSpd_rpm/1 -> MTQR_SL5REDUTqIncSR_Z_Nm/2
  VDHP_ActAPSPosn_pct/1 -> MTQR_SL5REDUTqIncSR_Z_Nm/1
  VTQR_SportTqRrIncGain_c/1 -> Product/2
  MTQR_SL5REDUTqIncSR_Z_Nm/1 -> Product/1
  Product/1 -> VTQR_SL5REDUTqIncSR_Nm/1

== system tqr/TQR/Determine Torque Request/TorqueArbitrament/TorqueSmooth/Rear wheel rate limit determination/VTQR_SPORTREDURateLimitInc_Nm/OPD ==
  VDHP_ActAPSPosn_pct : Inport
  VTQD_TqTargetShaftSpd_rpm : Inport  Port=2
  VTQR_SportTqRrIncGain_c : Inport  Port=3
  Action Port : ActionPort
  MTQR_SOPDREDUTqIncSR_Z_Nm : Lookup_n-D  BreakpointsForDimension1=ATQR_SL1FEDUTqIncSR_Y_pct  BreakpointsForDimension2=ATQR_SL1FEDUTqIncSR_X_rpm  Table=MTQR_SOPDREDUTqIncSR_Z_Nm  ExtrapMethod=Clip  InternalRulePriority=Speed  RndMeth=Simplest  InputSameDT=on
      settings: InputPortMap=u0,u1
  Product : Product
  VTQR_SOPDREDUTqIncSR_Nm : Outport
  wires:
  VTQD_TqTargetShaftSpd_rpm/1 -> MTQR_SOPDREDUTqIncSR_Z_Nm/2
  VDHP_ActAPSPosn_pct/1 -> MTQR_SOPDREDUTqIncSR_Z_Nm/1
  VTQR_SportTqRrIncGain_c/1 -> Product/2
  MTQR_SOPDREDUTqIncSR_Z_Nm/1 -> Product/1
  Product/1 -> VTQR_SOPDREDUTqIncSR_Nm/1
